simulink model "Project_01"  (R2014b)
settings: Solver=ode23tb  StartTime=0.0  StopTime=10.0  RelTol=1e-3
undefined symbols (not defined in the file): sigbuilder_block
libraries: powerlib x27, powerlib_meascontrol x2
settings Model: Creator=LENOVO  LastModifiedBy=LENOVO

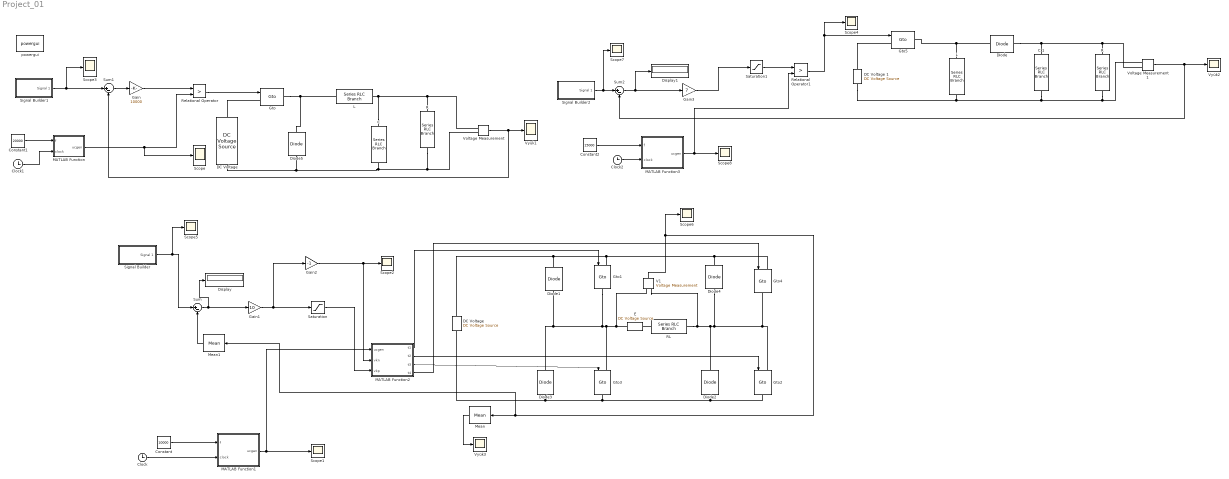
== system Project_01 ==
  " L" : powerlib/Elements/Series RLC Branch  LConnTagsString=__new0  RConnTagsString=__new0  BranchType=L  Resistance=1  Inductance=3*(1e-4)  SetiL0=off  InitialCurrent=0  Capacitance=1e-6  Setx0=off  InitialVoltage=0  Measurements=None
  " E" : powerlib/Electrical Sources/DC Voltage Source  Amplitude=50  Measurements=None
  " R" : powerlib/Elements/Series RLC Branch  LConnTagsString=__new0  RConnTagsString=__new0  BranchType=R  Resistance=100  Inductance=1e-3  SetiL0=off  InitialCurrent=0  Capacitance=1e-6  Setx0=off  InitialVoltage=0  Measurements=None
  C 1 : powerlib/Elements/Series RLC Branch  LConnTagsString=__new0  RConnTagsString=__new0  BranchType=C  Resistance=1  Inductance=1e-3  SetiL0=off  InitialCurrent=0  Capacitance=(1e-6)*250  Setx0=off  InitialVoltage=0  Measurements=None
  "C " : powerlib/Elements/Series RLC Branch  LConnTagsString=__new0  RConnTagsString=__new0  BranchType=C  Resistance=1  Inductance=1e-3  SetiL0=off  InitialCurrent=0  Capacitance=(1e-6)*470  Setx0=off  InitialVoltage=0  Measurements=None
  Clock : Clock
  Clock1 : Clock
  Clock2 : Clock
  Constant : Constant  Value=10000
  Constant1 : Constant  Value=20000
  Constant2 : Constant  Value=15000
  "DC Voltage " : powerlib/Electrical Sources/DC Voltage Source  Amplitude=15  Measurements=None
  "DC Voltage " : powerlib/Electrical Sources/DC Voltage Source  Amplitude=270  Measurements=None
  DC Voltage 1 : powerlib/Electrical Sources/DC Voltage Source  Amplitude=15  Measurements=None
  Diode : powerlib/Power Electronics/Diode  Ron=0.01  Lon=0.01  Vf=1  IC=0  UseSnubber=off  Rs=5000  Cs=250e-2  Measurements=off
  Diode{1..4} (4 alike) : powerlib/Power Electronics/Diode  Ron=0.001  Lon=0  Vf=0.8  IC=0  UseSnubber=off  Rs=500  Cs=250e-9  Measurements=off
  Diode5 : powerlib/Power Electronics/Diode  Ron=0.01  Lon=1e-4  Vf=0.8  IC=0  UseSnubber=off  Rs=10000  Cs=1e-4  Measurements=off
  Display : Display
  Display1 : Display
  Gain : Gain  Gain=10000
  Gain1 : Gain  Gain=10
  Gain2 : Gain  Gain=-1
  Gain3 : Gain  Gain=7
  Gto : powerlib/Power Electronics/Gto  Ron=0.01  Lon=0.001  Vf=0.8  Tf=10e-6  Tt=20e-6  IC=0  Rs=10000  Cs=1e-5  Measurements=off
  Gto{1..4} (4 alike) : powerlib/Power Electronics/Gto  Ron=0.01  Lon=0.00001  Vf=0.8  Tf=10e-6  Tt=20e-7  IC=0  Rs=10000  Cs=inf  Measurements=off
  Gto5 : powerlib/Power Electronics/Gto  Ron=0.01  Lon=0.01  Vf=0.8  Tf=10e-6  Tt=20e-7  IC=0  Rs=10000  Cs=inf  Measurements=off
  L : powerlib/Elements/Series RLC Branch  LConnTagsString=__new0  RConnTagsString=__new0  BranchType=L  Resistance=1  Inductance=1e-4  SetiL0=off  InitialCurrent=0  Capacitance=1e-6  Setx0=off  InitialVoltage=0  Measurements=None
  MATLAB Function : MATLAB Function  TreatAsAtomicUnit=on
  MATLAB Function1 : MATLAB Function  TreatAsAtomicUnit=on
  MATLAB Function2 : MATLAB Function  TreatAsAtomicUnit=on
  MATLAB Function3 : MATLAB Function  TreatAsAtomicUnit=on
  Mean : powerlib_meascontrol/Measurements/Mean  Freq=50  Vinit=0  Ts=0
  Mean1 : powerlib_meascontrol/Measurements/Mean  Freq=50  Vinit=0  Ts=0
  R : powerlib/Elements/Series RLC Branch  LConnTagsString=__new0  RConnTagsString=__new0  BranchType=R  Resistance=25  Inductance=1e-3  SetiL0=off  InitialCurrent=0  Capacitance=1e-6  Setx0=off  InitialVoltage=0  Measurements=None
  RL : powerlib/Elements/Series RLC Branch  LConnTagsString=__new0  RConnTagsString=__new0  BranchType=RL  Resistance=1  Inductance=1e-3  SetiL0=off  InitialCurrent=0  Capacitance=1e-6  Setx0=off  InitialVoltage=0  Measurements=None
  Relational Operator : RelationalOperator  Operator=>  OutDataTypeStr=boolean
  Relational Operator1 : RelationalOperator  Operator=>  OutDataTypeStr=boolean
  Saturation : Saturate  UpperLimit=1  LowerLimit=0
  Saturation1 : Saturate
  Scope{,1..8} (9 alike) : Scope
      Scope settings: YMin=0  YMax=12  SaveName=ScopeData3
      Scope1 settings: TimeRange=10  YMin=-1  YMax=2
      Scope2 settings: TimeRange=10  YMin=-500000  YMax=2e+06  SaveName=ScopeData2
      Scope3 settings: YMin=0  YMax=13  SaveName=ScopeData4
      Scope4 settings: YMin=0  YMax=30  SaveName=ScopeData8
      Scope5 settings: TimeRange=10  YMin=0  YMax=300  SaveName=ScopeData5
      Scope6 settings: TimeRange=10  YMin=-300  YMax=300  SaveName=ScopeData6
      Scope7 settings: YMin=0  YMax=30  SaveName=ScopeData9
      Scope8 settings: YMin=-1  YMax=1  SaveName=ScopeData10
  Signal Builder : Subsystem  Tag=STV Subsys  LoadFcn=sigbuilder_block('load');  StartFcn=sigbuilder_block('start');  StopFcn=sigbuilder_block('stop');  ClipboardFcn=sigbuilder_block('clipboard');  mask(Sigbuilder block){}
      mask help: Simulink:masks:SigbuilderBlock_MD
      mask init:
      | if ~strcmp(get_param(bdroot(gcbh),'SimulationStatus'),'stopped') tuvar = sigbuilder_block('maskInit'); end
      settings: CopyFcn=sigbuilder_block('copy');  DeleteFcn=sigbuilder_block('delete');  ModelCloseFcn=sigbuilder_block('modelClose');  PreSaveFcn=sigbuilder_block('preSave');  PauseFcn=sigbuilder_block('pause');  ContinueFcn=sigbuilder_block('continue');  NameChangeFcn=sigbuilder_block('namechange');  OpenFcn=sigbuilder_block('open',[437.6 199.2 550.4 400 ]);  CloseFcn=sigbuilder_block('close');
      mask Display: plot(0, 0, 100, 100,[2, 2, 32, 32, 2], [68, 8, 8, 68, 68],[32, 2], [38, 38], [32, 19, 2],[53, 60, 44], [32, 17, 17, 2],[16, 16, 31, 31]);txt = getActiveGroup(gcbh);text(2, 100, txt,'verticalAlignment', 'top');
  Signal Builder1 : Subsystem  Tag=STV Subsys  LoadFcn=sigbuilder_block('load');  StartFcn=sigbuilder_block('start');  StopFcn=sigbuilder_block('stop');  ClipboardFcn=sigbuilder_block('clipboard');  mask(Sigbuilder block){}
      mask help: Simulink:masks:SigbuilderBlock_MD
      mask init:
      | if ~strcmp(get_param(bdroot(gcbh),'SimulationStatus'),'stopped') tuvar = sigbuilder_block('maskInit'); end
      settings: CopyFcn=sigbuilder_block('copy');  DeleteFcn=sigbuilder_block('delete');  ModelCloseFcn=sigbuilder_block('modelClose');  PreSaveFcn=sigbuilder_block('preSave');  PauseFcn=sigbuilder_block('pause');  ContinueFcn=sigbuilder_block('continue');  NameChangeFcn=sigbuilder_block('namechange');  OpenFcn=sigbuilder_block('open',[437.6 199.2 550.4 400 ]);  CloseFcn=sigbuilder_block('close');
      mask Display: plot(0, 0, 100, 100,[2, 2, 32, 32, 2], [68, 8, 8, 68, 68],[32, 2], [38, 38], [32, 19, 2],[53, 60, 44], [32, 17, 17, 2],[16, 16, 31, 31]);txt = getActiveGroup(gcbh);text(2, 100, txt,'verticalAlignment', 'top');
  Signal Builder2 : Subsystem  Tag=STV Subsys  LoadFcn=sigbuilder_block('load');  StartFcn=sigbuilder_block('start');  StopFcn=sigbuilder_block('stop');  ClipboardFcn=sigbuilder_block('clipboard');  mask(Sigbuilder block){}
      mask help: Simulink:masks:SigbuilderBlock_MD
      mask init:
      | if ~strcmp(get_param(bdroot(gcbh),'SimulationStatus'),'stopped') tuvar = sigbuilder_block('maskInit'); end
      settings: CopyFcn=sigbuilder_block('copy');  DeleteFcn=sigbuilder_block('delete');  ModelCloseFcn=sigbuilder_block('modelClose');  PreSaveFcn=sigbuilder_block('preSave');  PauseFcn=sigbuilder_block('pause');  ContinueFcn=sigbuilder_block('continue');  NameChangeFcn=sigbuilder_block('namechange');  OpenFcn=sigbuilder_block('open',[437.6 199.2 550.4 400 ]);  CloseFcn=sigbuilder_block('close');
      mask Display: plot(0, 0, 100, 100,[2, 2, 32, 32, 2], [68, 8, 8, 68, 68],[32, 2], [38, 38], [32, 19, 2],[53, 60, 44], [32, 17, 17, 2],[16, 16, 31, 31]);txt = getActiveGroup(gcbh);text(2, 100, txt,'verticalAlignment', 'top');
  Sum : Sum  Inputs=|+-
  Sum1 : Sum  Inputs=|+-
  Sum2 : Sum  Inputs=|+-
  V1 : powerlib/Measurements/Voltage Measurement  PhasorSimulation=off  OutputType=Complex  PSBequivalent=0
  Voltage Measurement : powerlib/Measurements/Voltage Measurement  PhasorSimulation=off  OutputType=Complex  PSBequivalent=0
  Voltage Measurement1 : powerlib/Measurements/Voltage Measurement  PhasorSimulation=off  OutputType=Complex  PSBequivalent=0
  Vyük1 : Scope
      settings: TickLabels=on  TimeRange=10  YMin=0  YMax=13  SaveName=ScopeData7  MaxDataPoints=50000000
  "Vyük2 " : Scope
      settings: TimeRange=10  YMin=0  YMax=45  SaveName=ScopeData11
  Vyük3 : Scope
      settings: TimeRange=10  YMin=-200  YMax=300
  powergui : powerlib/powergui  Priority=1  SimulationMode=Discrete  SolverType=Tustin  SampleTime=1e-006  frequency=60  SPID=off  DisableSnubberDevices=off  DisableRonSwitches=off  DisableVfSwitches=off  SwTol=0  DisplayEquations=off  Interpol=off  methode=off  Ts=100  frequencyindice=0  Pbase=100e6  ErrMax=1e-4  Iterations=50  UnitsV=kV  UnitsW=MW  FunctionMessages=off  echomessages=off  HookPort=off  EnableUseOfTLC=off  x0status=blocks  RestoreLinks=warning  ResistiveCurrentMeasurement=off  Frange=[0:2:500]  Ylog=off  Xlog=on  ShowGrid=off  save=off  variable=ZData  structure=0  ZoomFFT=off  StartTime=0.0  cycles=1  DisplayStyle=1  fundamental=60  FreqAxis=off  MaxFrequency=1000  frequencyindicesteady=1  RmsSteady=1  display=off
  wires:
  Signal Builder/1(Signal 1) -> Scope5/1, Sum/1
  Clock/1 -> MATLAB Function1/2(clock)
  Constant/1 -> MATLAB Function1/1(f)
  Sum/1 -> Gain1/1, Display/1
  Gain2/1 -> Scope2/1, MATLAB Function2/2(vkn)
  Gain1/1 -> Gain2/1, Saturation/1
  V1/1 -> Mean1/1, Mean/1, Scope6/1
  Mean1/1 -> Sum/2
  Saturation/1 -> MATLAB Function2/3(vkp)
  Mean/1 -> Vyük3/1
  MATLAB Function1/1(ucgen) -> MATLAB Function2/1(ucgen), Scope1/1
  MATLAB Function2/1(t1) -> Gto1/1
  MATLAB Function2/2(t2) -> Gto2/1
  MATLAB Function2/3(t3) -> Gto3/1
  MATLAB Function2/4(t4) -> Gto4/1
  Clock1/1 -> MATLAB Function/2(clock)
  Constant1/1 -> MATLAB Function/1(f)
  Voltage Measurement/1 -> Vyük1/1, Sum1/2
  Signal Builder1/1(Signal 1) -> Scope3/1, Sum1/1
  Sum1/1 -> Gain/1
  Relational Operator/1 -> Gto/1
  MATLAB Function/1(ucgen) -> Scope/1, Relational Operator/2
  Gain/1 -> Relational Operator/1
  Voltage Measurement1/1 -> Sum2/2, "Vyük2 "/1
  Signal Builder2/1(Signal 1) -> Scope7/1, Sum2/1
  Sum2/1 -> Display1/1, Gain3/1
  Relational Operator1/1 -> Scope4/1, Gto5/1
  Saturation1/1 -> Relational Operator1/1
  Constant2/1 -> MATLAB Function3/1(f)
  Clock2/1 -> MATLAB Function3/2(clock)
  Gain3/1 -> Saturation1/1
  MATLAB Function3/1(ucgen) -> Relational Operator1/2, Scope8/1
  connections:
  RL/LConn1 -- " E"/LConn1
  Diode4/LConn1 -- RL/RConn1 -- V1/LConn2 -- Diode2/RConn1 -- Gto2/LConn1 -- Gto4/RConn1
  Diode3/LConn1 -- Gto2/RConn1 -- Diode2/LConn1 -- Gto3/RConn1 -- "DC Voltage "/LConn1
  "DC Voltage "/RConn1 -- Gto4/LConn1 -- Diode4/RConn1 -- Gto1/LConn1 -- Diode1/RConn1
  Diode3/RConn1 -- Gto3/LConn1 -- V1/LConn1 -- " E"/RConn1 -- Gto1/RConn1 -- Diode1/LConn1
  Gto/RConn1 -- Diode5/RConn1 -- L/LConn1
  "C "/LConn1 -- L/RConn1 -- Voltage Measurement/LConn1 -- R/LConn1
  "C "/RConn1 -- "DC Voltage "/LConn1 -- Diode5/LConn1 -- R/RConn1 -- Voltage Measurement/LConn2
  "DC Voltage "/RConn1 -- Gto/LConn1
  Diode/LConn1 -- C 1/LConn1 -- " R"/LConn1 -- Voltage Measurement1/LConn2
  Gto5/RConn1 -- " L"/LConn1 -- Diode/RConn1
  " L"/RConn1 -- DC Voltage 1/LConn1 -- " R"/RConn1 -- Voltage Measurement1/LConn1 -- C 1/RConn1
  DC Voltage 1/RConn1 -- Gto5/LConn1

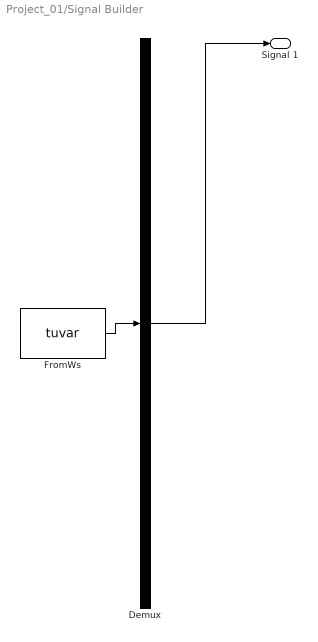
== system Project_01/Signal Builder ==
  Demux : Demux  Tag=STV Demux  Outputs=1
  FromWs : FromWorkspace  Tag=STV FromWs  VariableName=tuvar  SampleTime=0
      SigBuilderData=|
      | common.afterFinalStr = 'Extrapolate'
      | common.sampleTime = 0
      | dataSet.timeRange = [0 10]
      | dataSet.name = 'Group 1'
      | sbobj.Groups.Name = 'Group 1'
      | sbobj.Groups.Signals.Name = 'Signal 1'
      | sbobj.Groups.Signals.XData = [0 0.05 0.05 1 1.05 2 2 2.05 3 3.05 4 4 4.05 5 5.05 6 6 7 7.05 8 8 8.05 9 9.05 10]
      | sbobj.Groups.Signals.YData = [50 49.9 50 50 50 50 150 150 150 150 150 250 250 250 250 250 50 50 50 50 -150 -150 -150 -150 -150]
  Signal 1 : Outport  Tag=STV Outport
  wires:
  Demux/1 -> Signal 1/1
  FromWs/1 -> Demux/1

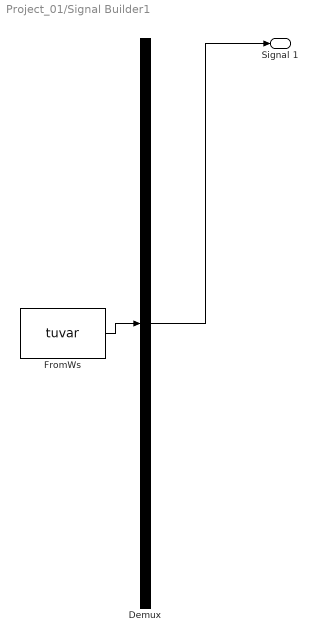
== system Project_01/Signal Builder1 ==
  Demux : Demux  Tag=STV Demux  Outputs=1
  FromWs : FromWorkspace  Tag=STV FromWs  VariableName=tuvar  SampleTime=0
      SigBuilderData=|
      | common.afterFinalStr = 'Extrapolate'
      | common.sampleTime = 0
      | dataSet.timeRange = [0 10]
      | dataSet.name = 'Group 1'
      | sbobj.Groups.Name = 'Group 1'
      | sbobj.Groups.Signals.Name = 'Signal 1'
      | sbobj.Groups.Signals.XData = [0 3 3 4 6 6 8 8 10]
      | sbobj.Groups.Signals.YData = [12 12 6 6 6 4 4 8 8]
  Signal 1 : Outport  Tag=STV Outport
  wires:
  Demux/1 -> Signal 1/1
  FromWs/1 -> Demux/1

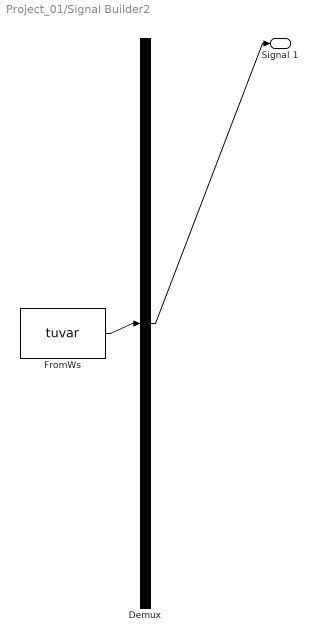
== system Project_01/Signal Builder2 ==
  Demux : Demux  Tag=STV Demux  Outputs=1
  FromWs : FromWorkspace  Tag=STV FromWs  VariableName=tuvar  SampleTime=0
      SigBuilderData=|
      | common.afterFinalStr = 'Extrapolate'
      | common.sampleTime = 0
      | dataSet.timeRange = [0 10]
      | dataSet.name = 'Group 1'
      | sbobj.Groups.Name = 'Group 1'
      | sbobj.Groups.Signals.Name = 'Signal 1'
      | sbobj.Groups.Signals.XData = [0 1 1 1.5 2.5 3 3 3.5 4 4.5 5 5 5.5 6 6.5 7 7 7.5 7.5 8 8.5 9 9 9.5 10]
      | sbobj.Groups.Signals.YData = [15 15 10 10 10 10 20 20 20 20 20 25 25 25 25 25 5 5 5.05 5 5 5 10 10 10]
  Signal 1 : Outport  Tag=STV Outport
  wires:
  Demux/1 -> Signal 1/1
  FromWs/1 -> Demux/1

== matlab function Project_01/MATLAB Function1 ==
  data: f input; ucgen output; clock input
function ucgen= fcn(f,clock)
%#codegen
genlik=1;
ucgen=0;
carpan=1;
p=1/(2*f);
tepe_zaman=p/2;
t=mod(clock,2*p);
zaman=mod(clock,p);
if(t<p)
    carpan=-1;
else
    carpan=1;
end
if (zaman >= tepe_zaman)
    ucgen=carpan*((genlik/tepe_zaman)*(p-zaman));
else
    ucgen=carpan*((genlik/tepe_zaman)*zaman);
end
return

== matlab function Project_01/MATLAB Function2 ==
  data: ucgen input; vkn input; vkp input; t1 output; t2 output; t3 output; t4 output
function [t1,t2,t3,t4]= tk(ucgen,vkn,vkp)
t1=0;
t2=0;
t3=0;
t4=0;
if(vkp>=ucgen)
    t1=1;
end
if (vkp<ucgen)
    t3=1;
end
if(vkn>=ucgen)
    t4=1;
end  
if(vkn<ucgen)
    t2=1;
end
return

== matlab function Project_01/MATLAB Function ==
  data: f input; ucgen output; clock input
function ucgen= fcn(f,clock)
%#codegen
genlik=1;
ucgen=0;
carpan=1;
p=1/(2*f);
tepe_zaman=p/2;
t=mod(clock,2*p);
zaman=mod(clock,p);
if(t<p)
    carpan=-1;
else
    carpan=1;
end
if (zaman >= tepe_zaman)
    ucgen=carpan*((genlik/tepe_zaman)*(p-zaman));
else
    ucgen=carpan*((genlik/tepe_zaman)*zaman);
end
return

== matlab function Project_01/MATLAB Function3 ==
  data: f input; ucgen output; clock input
function ucgen= fcn(f,clock)
%#codegen
genlik=1;
ucgen=0;
carpan=1;
p=1/(2*f);
tepe_zaman=p/2;
t=mod(clock,2*p);
zaman=mod(clock,p);
if(t<p)
    carpan=-1;
else
    carpan=1;
end
if (zaman >= tepe_zaman)
    ucgen=carpan*((genlik/tepe_zaman)*(p-zaman));
else
    ucgen=carpan*((genlik/tepe_zaman)*zaman);
end
return
